simulink model "IEEE33BusTestSystem_DG_Control_IMC"  (R2019a)
settings: Solver=ode23t  StartTime=0.0  StopTime=20  FixedStep=5e-5  RelTol=1e-3
values from neighbouring files (symbols this model uses):
  du_n = 500    [IEEE33BusSystem_Control_Sim.m]    (also in IEEE33BusSystem_Control_Sim_nq3.m; IEEE33BusSystem_Control_Sim_nq5.m; IEEE33BusSystem_Ident.m; IEEE33BusSystem_Sim_compare.m)
  dy_n = 0.03    [IEEE33BusSystem_Control_Sim.m]    (also in IEEE33BusSystem_Control_Sim_nq3.m; IEEE33BusSystem_Control_Sim_nq5.m; IEEE33BusSystem_Ident.m; IEEE33BusSystem_Sim_compare.m)
  P_dg0 = 300*ones(1,6)    [IEEE33BusSystem_Control_Sim.m]    (also in IEEE33BusSystem_Control_Sim_nq3.m; IEEE33BusSystem_Control_Sim_nq5.m; IEEE33BusSystem_Ident.m; IEEE33BusSystem_op.m)
  P_dgf = 100*ones(1,6)    [IEEE33BusSystem_Control_Sim.m]    (also in IEEE33BusSystem_Control_Sim_nq3.m; IEEE33BusSystem_Control_Sim_nq5.m; IEEE33BusSystem_op.m = 300*ones(1,6); Kimc_d1_sce1-0.mat = [100 100 100 100 100 100])
  Q_dg0 = zeros(1,6)    [IEEE33BusSystem_Control_Sim.m]    (also in IEEE33BusSystem_Control_Sim_nq3.m; IEEE33BusSystem_Control_Sim_nq5.m; IEEE33BusSystem_Ident.m; IEEE33BusSystem_op.m)
  Tp = 500e-3    (= 0.5)    [IEEE33BusSystem.m]    (also in Kimc_d1_sce1-0.mat = 0.05; Kimc_d1_sce1-1.mat = 0.05; Kimc_d1_sce1-2.mat = 0.05; Kimc_d1_sce1-3.mat = 0.05)
  tPdg = 10*ones(1,6)    [IEEE33BusSystem_Control_Sim.m]    (also in IEEE33BusSystem_Control_Sim_nq3.m; IEEE33BusSystem_Control_Sim_nq5.m; IEEE33BusSystem_op.m = 0.5*ones(1,6); Kimc_d1_sce1-0.mat = [10 10 10 10 10 10])
  Tq = 50e-3    (= 0.05)    [IEEE33BusSystem.m]    (also in Kimc_d1_sce1-0.mat; Kimc_d1_sce1-1.mat; Kimc_d1_sce1-2.mat; Kimc_d1_sce1-3.mat)
  Ts = 0.005    [IEEE33BusSystem_Control_Sim.m]    (also in IEEE33BusSystem_Control_Sim_nq3.m; IEEE33BusSystem_Control_Sim_nq5.m; IEEE33BusSystem_Sim_compare.m = tout_d(2)-tout_d(1); IEEE33BusSystem_op.m)
  tsp = 3*ones(1,6)    [IEEE33BusSystem_Control_Sim.m]    (also in IEEE33BusSystem_Control_Sim_nq3.m; IEEE33BusSystem_Control_Sim_nq5.m; Kimc_d1_sce1-0.mat = [3 3 3 3 3 3]; Kimc_d1_sce1-1.mat = [3 3 3 3 3 3])
  v0 = ones(1,33)    [IEEE33BusSystem_Control_Sim.m]    (also in IEEE33BusSystem_Control_Sim_nq3.m; IEEE33BusSystem_Control_Sim_nq5.m; IEEE33BusSystem_Ident.m; IEEE33BusSystem_op.m)
  V_0 = v0_sim(CVs_sel)    [IEEE33BusSystem_Control_Sim.m]    (also in IEEE33BusSystem_Control_Sim_nq3.m = [v0_sim(14), v0_sim(18), v0_sim(21), v0_sim(25), v0_sim(30),; IEEE33BusSystem_Control_Sim_nq5.m = [v0_sim(14), v0_sim(18), v0_sim(21), v0_sim(25), v0_sim(30),; IEEE33BusSystem_Ident.m; IEEE33BusSystem_op.m = [v0(14), v0(18), v0(21), v0(25), v0(30), v0(33)])
  Vsp = V_0    [IEEE33BusSystem_Control_Sim.m]    (also in IEEE33BusSystem_Control_Sim_nq3.m; IEEE33BusSystem_Control_Sim_nq5.m; Kimc_d1_sce1-0.mat = [0.9549 0.956 0.9966 0.9787 0.9486 0.9462]; Kimc_d1_sce1-1.mat = [0.9549 0.956 0.9966 0.9787 0.9486 0.9462])
libraries: powerlib x160, powerlib_meascontrol x33, cstblocks x2
(part 2 of 4)

== system IEEE33BusTestSystem_DG_Control_IMC/ADN/Bus_13 ==
  Bus Load 13 : powerlib/Elements/Three-Phase Series RLC Load  LConnTagsString=A|B|C  Configuration=Y (grounded)  NominalVoltage=(12660)*v0(13)  Vabc=[1e3 1e3 1e3]  Vabcp=[1e3 1e3 1e3]  NominalFrequency=50  UnbalancedPower=off  ActivePower=60e3  InductivePower=35e3  CapacitivePower=0  Pabc=[10e3 9e3 11e3]  QLabc=[100 90 110]  QCabc=[100 90 110]  Pabcp=[10e3 9e3 11e3]  QLabcp=[100 90 110]  QCabcp=[100 90 110]  Measurements=None  LoadType=constant PQ
      settings: SourceProductName=Simscape Electrical
  Bus_13 : powerlib/Measurements/Three-Phase V-I Measurement  VoltageMeasurement=phase-to-phase  SetLabelV=on  LabelV=v13_pu  Vpu=off  VpuLL=on  CurrentMeasurement=yes  SetLabelI=on  LabelI=I1213_pu  Ipu=off  Pbase=100e6  Vbase=12660  OutputType=Complex  PhasorSimulation=on  PSBequivalent=0
      settings: SourceProductName=Simscape Electrical
  CB3-2 : powerlib/Elements/Three-Phase Breaker  InitialState=open  SwitchA=on  SwitchB=on  SwitchC=on  SwitchTimes="[1/60  5/60]"  External=on  BreakerResistance=0.01  SnubberResistance=1e6  SnubberCapacitance=inf  Measurements=None
      settings: SourceProductName=Simscape Electrical
  InPhaseA : PMIOPort  Side=Left
  InPhaseB : PMIOPort  Port=2  Side=Left
  InPhaseC : PMIOPort  Port=3  Side=Left
  OutPhaseA : PMIOPort  Port=4  Side=Right
  OutPhaseB : PMIOPort  Port=5  Side=Right
  OutPhaseC : PMIOPort  Port=6  Side=Right
  wires:
  [CB13to14] -> CB3-2/1
  connections:
  Bus Load 13/LConn1 -- CB3-2/LConn1 -- Bus_13/RConn1
  CB3-2/RConn3 -- OutPhaseC/RConn1
  Bus Load 13/LConn2 -- CB3-2/LConn2 -- Bus_13/RConn2
  Bus_13/RConn3 -- CB3-2/LConn3 -- Bus Load 13/LConn3
  CB3-2/RConn1 -- OutPhaseA/RConn1
  CB3-2/RConn2 -- OutPhaseB/RConn1
  InPhaseB/RConn1 -- Bus_13/LConn2
  Bus_13/LConn1 -- InPhaseA/RConn1
  InPhaseC/RConn1 -- Bus_13/LConn3

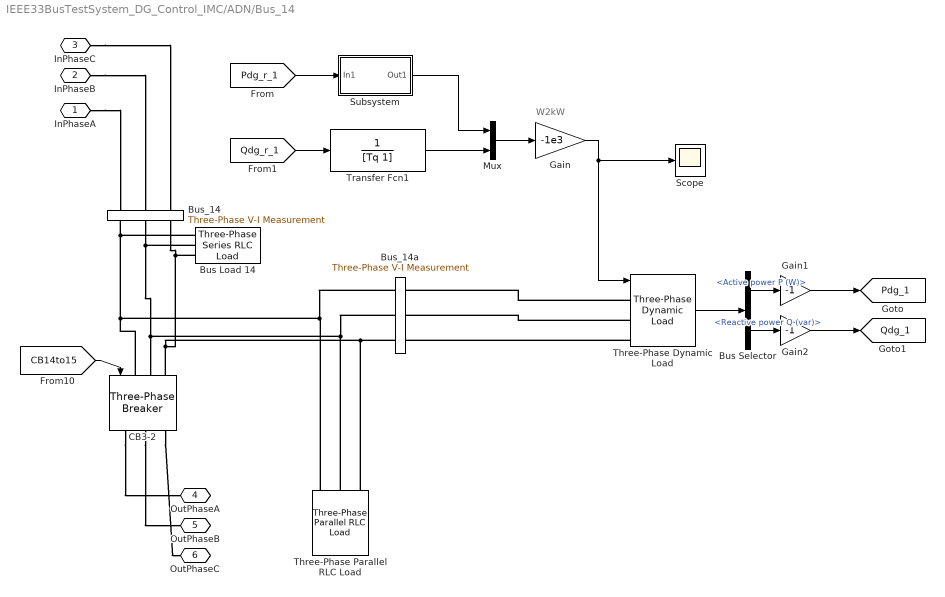
== system IEEE33BusTestSystem_DG_Control_IMC/ADN/Bus_14 ==
  note: W2kW
  Bus Load 14 : powerlib/Elements/Three-Phase Series RLC Load  LConnTagsString=A|B|C  Configuration=Y (grounded)  NominalVoltage=(12660)*v0(14)  Vabc=[1e3 1e3 1e3]  Vabcp=[1e3 1e3 1e3]  NominalFrequency=50  UnbalancedPower=off  ActivePower=120e3  InductivePower=80e3  CapacitivePower=0  Pabc=[10e3 9e3 11e3]  QLabc=[100 90 110]  QCabc=[100 90 110]  Pabcp=[10e3 9e3 11e3]  QLabcp=[100 90 110]  QCabcp=[100 90 110]  Measurements=None  LoadType=constant PQ
      settings: SourceProductName=Simscape Electrical
  Bus Selector : BusSelector  OutputSignals=Active power P (W),Reactive power Q (var)
  Bus_14 : powerlib/Measurements/Three-Phase V-I Measurement  VoltageMeasurement=phase-to-phase  SetLabelV=on  LabelV=v14_pu  Vpu=off  VpuLL=on  CurrentMeasurement=yes  SetLabelI=on  LabelI=I1314_pu  Ipu=off  Pbase=100e6  Vbase=12660  OutputType=Complex  PhasorSimulation=on  PSBequivalent=0
      settings: SourceProductName=Simscape Electrical
  Bus_14a : powerlib/Measurements/Three-Phase V-I Measurement  VoltageMeasurement=no  SetLabelV=off  LabelV=v14a_pu  Vpu=off  VpuLL=off  CurrentMeasurement=yes  SetLabelI=on  LabelI=I14a_pu  Ipu=off  Pbase=100e6  Vbase=500e3  OutputType=Complex  PhasorSimulation=on  PSBequivalent=0
      settings: SourceProductName=Simscape Electrical
  CB3-2 : powerlib/Elements/Three-Phase Breaker  InitialState=open  SwitchA=on  SwitchB=on  SwitchC=on  SwitchTimes="[1/60  5/60]"  External=on  BreakerResistance=0.01  SnubberResistance=1e6  SnubberCapacitance=inf  Measurements=None
      settings: SourceProductName=Simscape Electrical
  Gain : Gain  Gain=-1e3
  Gain1 : Gain  Gain=-1
  Gain2 : Gain  Gain=-1
  Mux : Mux  Inputs=2
  Scope : Scope
  Subsystem : Subsystem
  Three-Phase Dynamic Load : powerlib/Elements/Three-Phase Dynamic Load  NominalVoltage=[ 12660 50 ]  ActiveReactivePowers=[-P_dg0(1) Q_dg0(1)]*1e3  PositiveSequence=[V_0(1) 0]  ExternalControl=on  NpNq=[1.3 2]  TimeConstants="[0  0  0  0]"  MinimumVoltage=0.7  Tfilter=1e-4  LoadFlowParameters=[4,0,0,0,0]
      settings: SourceProductName=Simscape Electrical  SourceProductBaseCode=PS
  Three-Phase Parallel RLC Load : powerlib/Elements/Three-Phase Parallel RLC Load  LConnTagsString=A|B|C  Configuration=Y (grounded)  NominalVoltage=12660  Vabc=[1e3 1e3 1e3]  Vabcp=[1e3 1e3 1e3]  NominalFrequency=50  UnbalancedPower=off  ActivePower=0.01  InductivePower=0  CapacitivePower=0  Pabc=[10e3 9e3 11e3]  QLabc=[100 90 110]  QCabc=[100 90 110]  Pabcp=[10e3 9e3 11e3]  QLabcp=[100 90 110]  QCabcp=[100 90 110]  Measurements=None  LoadType=constant Z
      settings: SourceProductName=Simscape Electrical
  Transfer Fcn1 : TransferFcn  Denominator=[Tq 1]
  InPhaseA : PMIOPort  Side=Left
  InPhaseB : PMIOPort  Port=2  Side=Left
  InPhaseC : PMIOPort  Port=3  Side=Left
  OutPhaseA : PMIOPort  Port=4  Side=Right
  OutPhaseB : PMIOPort  Port=5  Side=Right
  OutPhaseC : PMIOPort  Port=6  Side=Right
  tag scope: Pdg_1=global, Qdg_1=global
  wires:
  [CB14to15] -> CB3-2/1
  Mux/1 -> Gain/1
  Gain/1 -> Three-Phase Dynamic Load/1, Scope/1
  Three-Phase Dynamic Load/1 -> Bus Selector/1
  Subsystem/1(Out1) -> Mux/1
  Bus Selector/1 -> Gain1/1  "<Active power P (W)>"
  Bus Selector/2 -> Gain2/1  "<Reactive power Q (var)>"
  Gain1/1 -> [Pdg_1]
  Gain2/1 -> [Qdg_1]
  [Pdg_r_1] -> Subsystem/1(In1)
  [Qdg_r_1] -> Transfer Fcn1/1
  Transfer Fcn1/1 -> Mux/2
  connections:
  CB3-2/LConn1 -- Three-Phase Parallel RLC Load/LConn1 -- Bus_14a/RConn1 -- Bus Load 14/LConn1 -- Bus_14/RConn1
  CB3-2/RConn3 -- OutPhaseC/RConn1
  Bus_14/RConn3 -- Bus_14a/RConn3 -- Three-Phase Parallel RLC Load/LConn3 -- CB3-2/LConn3 -- Bus Load 14/LConn3
  CB3-2/RConn1 -- OutPhaseA/RConn1
  CB3-2/RConn2 -- OutPhaseB/RConn1
  InPhaseB/RConn1 -- Bus_14/LConn2
  InPhaseA/RConn1 -- Bus_14/LConn1
  InPhaseC/RConn1 -- Bus_14/LConn3
  Bus_14/RConn2 -- Bus Load 14/LConn2 -- Three-Phase Parallel RLC Load/LConn2 -- Bus_14a/RConn2 -- CB3-2/LConn2
  Three-Phase Dynamic Load/LConn1 -- Bus_14a/LConn1
  Three-Phase Dynamic Load/LConn2 -- Bus_14a/LConn2
  Three-Phase Dynamic Load/LConn3 -- Bus_14a/LConn3

== system IEEE33BusTestSystem_DG_Control_IMC/ADN/Bus_15 ==
  Bus Load 15 : powerlib/Elements/Three-Phase Series RLC Load  LConnTagsString=A|B|C  Configuration=Y (grounded)  NominalVoltage=(12660)*v0(15)  Vabc=[1e3 1e3 1e3]  Vabcp=[1e3 1e3 1e3]  NominalFrequency=50  UnbalancedPower=off  ActivePower=60e3  InductivePower=10e3  CapacitivePower=0  Pabc=[10e3 9e3 11e3]  QLabc=[100 90 110]  QCabc=[100 90 110]  Pabcp=[10e3 9e3 11e3]  QLabcp=[100 90 110]  QCabcp=[100 90 110]  Measurements=None  LoadType=constant PQ
      settings: SourceProductName=Simscape Electrical
  Bus_15 : powerlib/Measurements/Three-Phase V-I Measurement  VoltageMeasurement=phase-to-phase  SetLabelV=on  LabelV=v15_pu  Vpu=off  VpuLL=on  CurrentMeasurement=yes  SetLabelI=on  LabelI=I1415_pu  Ipu=off  Pbase=100e6  Vbase=12660  OutputType=Complex  PhasorSimulation=on  PSBequivalent=0
      settings: SourceProductName=Simscape Electrical
  CB3-2 : powerlib/Elements/Three-Phase Breaker  InitialState=open  SwitchA=on  SwitchB=on  SwitchC=on  SwitchTimes="[1/60  5/60]"  External=on  BreakerResistance=0.01  SnubberResistance=1e6  SnubberCapacitance=inf  Measurements=None
      settings: SourceProductName=Simscape Electrical
  InPhaseA : PMIOPort  Side=Left
  InPhaseB : PMIOPort  Port=2  Side=Left
  InPhaseC : PMIOPort  Port=3  Side=Left
  OutPhaseA : PMIOPort  Port=4  Side=Right
  OutPhaseB : PMIOPort  Port=5  Side=Right
  OutPhaseC : PMIOPort  Port=6  Side=Right
  InPhaseA1 : PMIOPort  Port=7  Side=Left
  InPhaseB1 : PMIOPort  Port=8  Side=Left
  InPhaseC1 : PMIOPort  Port=9  Side=Left
  wires:
  [CB15to16] -> CB3-2/1
  connections:
  Bus Load 15/LConn1 -- CB3-2/LConn1 -- Bus_15/RConn1
  CB3-2/RConn3 -- OutPhaseC/RConn1
  Bus Load 15/LConn2 -- CB3-2/LConn2 -- Bus_15/RConn2
  Bus Load 15/LConn3 -- CB3-2/LConn3 -- Bus_15/RConn3
  CB3-2/RConn1 -- OutPhaseA/RConn1
  CB3-2/RConn2 -- OutPhaseB/RConn1
  InPhaseA1/RConn1 -- InPhaseA/RConn1 -- Bus_15/LConn1
  InPhaseB1/RConn1 -- InPhaseB/RConn1 -- Bus_15/LConn2
  InPhaseC1/RConn1 -- InPhaseC/RConn1 -- Bus_15/LConn3

== system IEEE33BusTestSystem_DG_Control_IMC/ADN/Bus_16 ==
  Bus Load 16 : powerlib/Elements/Three-Phase Series RLC Load  LConnTagsString=A|B|C  Configuration=Y (grounded)  NominalVoltage=(12660)*v0(16)  Vabc=[1e3 1e3 1e3]  Vabcp=[1e3 1e3 1e3]  NominalFrequency=50  UnbalancedPower=off  ActivePower=60e3  InductivePower=20e3  CapacitivePower=0  Pabc=[10e3 9e3 11e3]  QLabc=[100 90 110]  QCabc=[100 90 110]  Pabcp=[10e3 9e3 11e3]  QLabcp=[100 90 110]  QCabcp=[100 90 110]  Measurements=None  LoadType=constant PQ
      settings: SourceProductName=Simscape Electrical
  Bus_16 : powerlib/Measurements/Three-Phase V-I Measurement  VoltageMeasurement=phase-to-phase  SetLabelV=on  LabelV=v16_pu  Vpu=off  VpuLL=on  CurrentMeasurement=yes  SetLabelI=on  LabelI=I1516_pu  Ipu=off  Pbase=100e6  Vbase=12660  OutputType=Complex  PhasorSimulation=on  PSBequivalent=0
      settings: SourceProductName=Simscape Electrical
  CB3-2 : powerlib/Elements/Three-Phase Breaker  InitialState=open  SwitchA=on  SwitchB=on  SwitchC=on  SwitchTimes="[1/60  5/60]"  External=on  BreakerResistance=0.01  SnubberResistance=1e6  SnubberCapacitance=inf  Measurements=None
      settings: SourceProductName=Simscape Electrical
  InPhaseA : PMIOPort  Side=Left
  InPhaseB : PMIOPort  Port=2  Side=Left
  InPhaseC : PMIOPort  Port=3  Side=Left
  OutPhaseA : PMIOPort  Port=4  Side=Right
  OutPhaseB : PMIOPort  Port=5  Side=Right
  OutPhaseC : PMIOPort  Port=6  Side=Right
  wires:
  [CB16to17] -> CB3-2/1
  connections:
  Bus_16/RConn1 -- CB3-2/LConn1 -- Bus Load 16/LConn1
  CB3-2/RConn3 -- OutPhaseC/RConn1
  Bus Load 16/LConn2 -- CB3-2/LConn2 -- Bus_16/RConn2
  Bus Load 16/LConn3 -- CB3-2/LConn3 -- Bus_16/RConn3
  CB3-2/RConn1 -- OutPhaseA/RConn1
  CB3-2/RConn2 -- OutPhaseB/RConn1
  InPhaseC/RConn1 -- Bus_16/LConn3
  InPhaseB/RConn1 -- Bus_16/LConn2
  InPhaseA/RConn1 -- Bus_16/LConn1

== system IEEE33BusTestSystem_DG_Control_IMC/ADN/Bus_17 ==
  Bus Load 17 : powerlib/Elements/Three-Phase Series RLC Load  LConnTagsString=A|B|C  Configuration=Y (grounded)  NominalVoltage=(12660)*v0(17)  Vabc=[1e3 1e3 1e3]  Vabcp=[1e3 1e3 1e3]  NominalFrequency=50  UnbalancedPower=off  ActivePower=60e3  InductivePower=20e3  CapacitivePower=0  Pabc=[10e3 9e3 11e3]  QLabc=[100 90 110]  QCabc=[100 90 110]  Pabcp=[10e3 9e3 11e3]  QLabcp=[100 90 110]  QCabcp=[100 90 110]  Measurements=None  LoadType=constant PQ
      settings: SourceProductName=Simscape Electrical
  Bus_17 : powerlib/Measurements/Three-Phase V-I Measurement  VoltageMeasurement=phase-to-phase  SetLabelV=on  LabelV=v17_pu  Vpu=off  VpuLL=on  CurrentMeasurement=yes  SetLabelI=on  LabelI=I1617_pu  Ipu=off  Pbase=100e6  Vbase=12660  OutputType=Complex  PhasorSimulation=on  PSBequivalent=0
      settings: SourceProductName=Simscape Electrical
  CB3-1 : powerlib/Elements/Three-Phase Breaker  InitialState=open  SwitchA=on  SwitchB=on  SwitchC=on  SwitchTimes="[1/60  5/60]"  External=on  BreakerResistance=0.01  SnubberResistance=1e6  SnubberCapacitance=inf  Measurements=None
      settings: SourceProductName=Simscape Electrical
  CB3-2 : powerlib/Elements/Three-Phase Breaker  InitialState=open  SwitchA=on  SwitchB=on  SwitchC=on  SwitchTimes="[1/60  5/60]"  External=on  BreakerResistance=0.01  SnubberResistance=1e6  SnubberCapacitance=inf  Measurements=None
      settings: SourceProductName=Simscape Electrical
  Step : Step  Time=2  Before=1  SampleTime=0
  InPhaseA : PMIOPort  Side=Left
  InPhaseB : PMIOPort  Port=2  Side=Left
  InPhaseC : PMIOPort  Port=3  Side=Left
  OutPhaseA : PMIOPort  Port=4  Side=Right
  OutPhaseB : PMIOPort  Port=5  Side=Right
  OutPhaseC : PMIOPort  Port=6  Side=Right
  wires:
  [CB17to18] -> CB3-2/1
  Step/1 -> CB3-1/1
  connections:
  CB3-2/LConn1 -- Bus_17/RConn1 -- CB3-1/RConn1
  CB3-2/RConn3 -- OutPhaseC/RConn1
  Bus_17/RConn2 -- CB3-1/RConn2 -- CB3-2/LConn2
  Bus_17/RConn3 -- CB3-1/RConn3 -- CB3-2/LConn3
  CB3-2/RConn1 -- OutPhaseA/RConn1
  CB3-2/RConn2 -- OutPhaseB/RConn1
  InPhaseA/RConn1 -- Bus_17/LConn1
  InPhaseB/RConn1 -- Bus_17/LConn2
  InPhaseC/RConn1 -- Bus_17/LConn3
  CB3-1/LConn1 -- Bus Load 17/LConn1
  CB3-1/LConn2 -- Bus Load 17/LConn2
  CB3-1/LConn3 -- Bus Load 17/LConn3

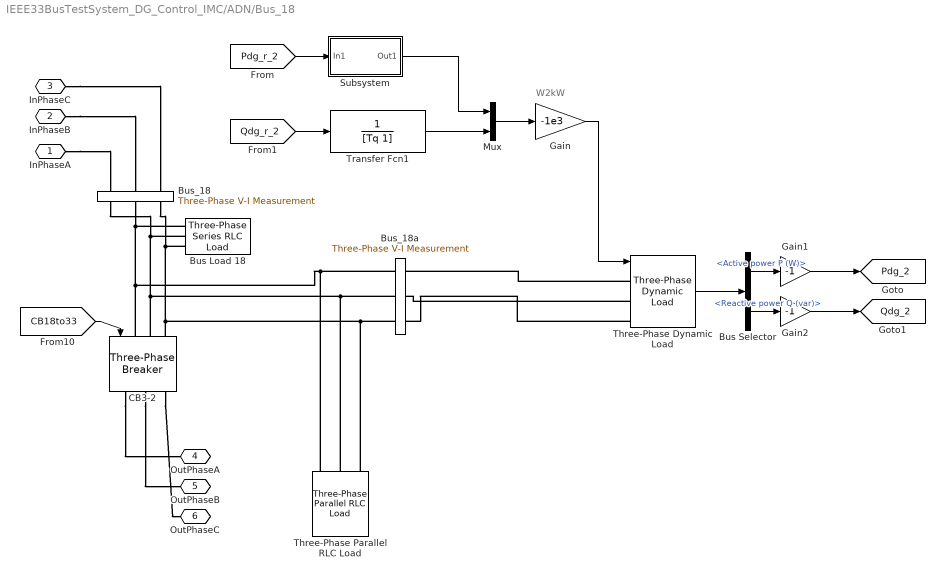
== system IEEE33BusTestSystem_DG_Control_IMC/ADN/Bus_18 ==
  note: W2kW
  Bus Load 18 : powerlib/Elements/Three-Phase Series RLC Load  LConnTagsString=A|B|C  Configuration=Y (grounded)  NominalVoltage=(12660)*v0(18)  Vabc=[1e3 1e3 1e3]  Vabcp=[1e3 1e3 1e3]  NominalFrequency=50  UnbalancedPower=off  ActivePower=90e3  InductivePower=40e3  CapacitivePower=0  Pabc=[10e3 9e3 11e3]  QLabc=[100 90 110]  QCabc=[100 90 110]  Pabcp=[10e3 9e3 11e3]  QLabcp=[100 90 110]  QCabcp=[100 90 110]  Measurements=None  LoadType=constant PQ
      settings: SourceProductName=Simscape Electrical
  Bus Selector : BusSelector  OutputSignals=Active power P (W),Reactive power Q (var)
  Bus_18 : powerlib/Measurements/Three-Phase V-I Measurement  VoltageMeasurement=phase-to-phase  SetLabelV=on  LabelV=v18_pu  Vpu=off  VpuLL=on  CurrentMeasurement=yes  SetLabelI=on  LabelI=I1718_pu  Ipu=off  Pbase=100e6  Vbase=12660  OutputType=Complex  PhasorSimulation=on  PSBequivalent=0
      settings: SourceProductName=Simscape Electrical
  Bus_18a : powerlib/Measurements/Three-Phase V-I Measurement  VoltageMeasurement=no  SetLabelV=off  LabelV=v14a_pu  Vpu=off  VpuLL=off  CurrentMeasurement=yes  SetLabelI=on  LabelI=I18a_pu  Ipu=off  Pbase=100e6  Vbase=500e3  OutputType=Complex  PhasorSimulation=on  PSBequivalent=0
      settings: SourceProductName=Simscape Electrical
  CB3-2 : powerlib/Elements/Three-Phase Breaker  InitialState=open  SwitchA=on  SwitchB=on  SwitchC=on  SwitchTimes="[1/60  5/60]"  External=on  BreakerResistance=0.01  SnubberResistance=1e6  SnubberCapacitance=inf  Measurements=None
      settings: SourceProductName=Simscape Electrical
  Gain : Gain  Gain=-1e3
  Gain1 : Gain  Gain=-1
  Gain2 : Gain  Gain=-1
  Mux : Mux  Inputs=2
  Subsystem : Subsystem
  Three-Phase Dynamic Load : powerlib/Elements/Three-Phase Dynamic Load  NominalVoltage=[ 12660 50 ]  ActiveReactivePowers=[-P_dg0(2) Q_dg0(2)]*1e3  PositiveSequence=[V_0(2) 0]  ExternalControl=on  NpNq=[1.3 2]  TimeConstants="[0  0  0  0]"  MinimumVoltage=0.7  Tfilter=1e-4  LoadFlowParameters=[4,0,0,0,0]
      settings: SourceProductName=Simscape Electrical  SourceProductBaseCode=PS
  Three-Phase Parallel RLC Load : powerlib/Elements/Three-Phase Parallel RLC Load  LConnTagsString=A|B|C  Configuration=Y (grounded)  NominalVoltage=12660  Vabc=[1e3 1e3 1e3]  Vabcp=[1e3 1e3 1e3]  NominalFrequency=50  UnbalancedPower=off  ActivePower=0.01  InductivePower=0  CapacitivePower=0  Pabc=[10e3 9e3 11e3]  QLabc=[100 90 110]  QCabc=[100 90 110]  Pabcp=[10e3 9e3 11e3]  QLabcp=[100 90 110]  QCabcp=[100 90 110]  Measurements=None  LoadType=constant Z
      settings: SourceProductName=Simscape Electrical
  Transfer Fcn1 : TransferFcn  Denominator=[Tq 1]
  InPhaseA : PMIOPort  Side=Left
  InPhaseB : PMIOPort  Port=2  Side=Left
  InPhaseC : PMIOPort  Port=3  Side=Left
  OutPhaseA : PMIOPort  Port=4  Side=Right
  OutPhaseB : PMIOPort  Port=5  Side=Right
  OutPhaseC : PMIOPort  Port=6  Side=Right
  tag scope: Pdg_2=global, Qdg_2=global
  wires:
  [CB18to33] -> CB3-2/1
  Subsystem/1(Out1) -> Mux/1
  Bus Selector/1 -> Gain1/1  "<Active power P (W)>"
  [Pdg_r_2] -> Subsystem/1(In1)
  Gain2/1 -> [Qdg_2]
  Bus Selector/2 -> Gain2/1  "<Reactive power Q (var)>"
  Mux/1 -> Gain/1
  Three-Phase Dynamic Load/1 -> Bus Selector/1
  Gain/1 -> Three-Phase Dynamic Load/1
  Gain1/1 -> [Pdg_2]
  [Qdg_r_2] -> Transfer Fcn1/1
  Transfer Fcn1/1 -> Mux/2
  connections:
  Bus_18/RConn1 -- Three-Phase Parallel RLC Load/LConn1 -- Bus_18a/RConn1 -- CB3-2/LConn1 -- Bus Load 18/LConn1
  CB3-2/RConn3 -- OutPhaseC/RConn1
  Bus Load 18/LConn2 -- Three-Phase Parallel RLC Load/LConn2 -- Bus_18a/RConn2 -- CB3-2/LConn2 -- Bus_18/RConn2
  Bus Load 18/LConn3 -- Three-Phase Parallel RLC Load/LConn3 -- Bus_18a/RConn3 -- CB3-2/LConn3 -- Bus_18/RConn3
  CB3-2/RConn1 -- OutPhaseA/RConn1
  CB3-2/RConn2 -- OutPhaseB/RConn1
  InPhaseA/RConn1 -- Bus_18/LConn1
  InPhaseB/RConn1 -- Bus_18/LConn2
  InPhaseC/RConn1 -- Bus_18/LConn3
  Three-Phase Dynamic Load/LConn1 -- Bus_18a/LConn1
  Three-Phase Dynamic Load/LConn3 -- Bus_18a/LConn3
  Three-Phase Dynamic Load/LConn2 -- Bus_18a/LConn2

== system IEEE33BusTestSystem_DG_Control_IMC/ADN/Bus_19 ==
  Bus Load 19 : powerlib/Elements/Three-Phase Series RLC Load  LConnTagsString=A|B|C  Configuration=Y (grounded)  NominalVoltage=(12660)*v0(19)  Vabc=[1e3 1e3 1e3]  Vabcp=[1e3 1e3 1e3]  NominalFrequency=50  UnbalancedPower=off  ActivePower=90e3  InductivePower=40e3  CapacitivePower=0  Pabc=[10e3 9e3 11e3]  QLabc=[100 90 110]  QCabc=[100 90 110]  Pabcp=[10e3 9e3 11e3]  QLabcp=[100 90 110]  QCabcp=[100 90 110]  Measurements=None  LoadType=constant PQ
      settings: SourceProductName=Simscape Electrical
  Bus_19 : powerlib/Measurements/Three-Phase V-I Measurement  VoltageMeasurement=phase-to-phase  SetLabelV=on  LabelV=v19_pu  Vpu=off  VpuLL=on  CurrentMeasurement=yes  SetLabelI=on  LabelI=I219_pu  Ipu=off  Pbase=100e6  Vbase=12660  OutputType=Complex  PhasorSimulation=on  PSBequivalent=0
      settings: SourceProductName=Simscape Electrical
  CB3-2 : powerlib/Elements/Three-Phase Breaker  InitialState=open  SwitchA=on  SwitchB=on  SwitchC=on  SwitchTimes="[1/60  5/60]"  External=on  BreakerResistance=0.01  SnubberResistance=1e6  SnubberCapacitance=inf  Measurements=None
      settings: SourceProductName=Simscape Electrical
  InPhaseA : PMIOPort  Side=Left
  InPhaseB : PMIOPort  Port=2  Side=Left
  InPhaseC : PMIOPort  Port=3  Side=Left
  OutPhaseA : PMIOPort  Port=4  Side=Right
  OutPhaseB : PMIOPort  Port=5  Side=Right
  OutPhaseC : PMIOPort  Port=6  Side=Right
  wires:
  [CB19to20] -> CB3-2/1
  connections:
  Bus_19/RConn1 -- CB3-2/LConn1 -- Bus Load 19/LConn1
  CB3-2/RConn3 -- OutPhaseC/RConn1
  Bus Load 19/LConn2 -- CB3-2/LConn2 -- Bus_19/RConn2
  Bus_19/RConn3 -- CB3-2/LConn3 -- Bus Load 19/LConn3
  CB3-2/RConn1 -- OutPhaseA/RConn1
  CB3-2/RConn2 -- OutPhaseB/RConn1
  Bus_19/LConn1 -- InPhaseA/RConn1
  InPhaseB/RConn1 -- Bus_19/LConn2
  InPhaseC/RConn1 -- Bus_19/LConn3

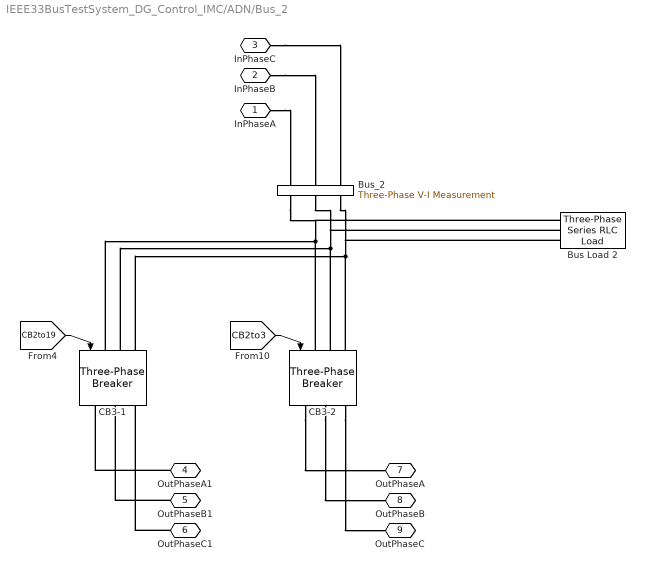
== system IEEE33BusTestSystem_DG_Control_IMC/ADN/Bus_2 ==
  Bus Load 2 : powerlib/Elements/Three-Phase Series RLC Load  LConnTagsString=A|B|C  Configuration=Y (grounded)  NominalVoltage=(12660)*v0(2)  Vabc=[1e3 1e3 1e3]  Vabcp=[1e3 1e3 1e3]  NominalFrequency=50  UnbalancedPower=off  ActivePower=100e3  InductivePower=60e3  CapacitivePower=0  Pabc=[10e3 9e3 11e3]  QLabc=[100 90 110]  QCabc=[100 90 110]  Pabcp=[10e3 9e3 11e3]  QLabcp=[100 90 110]  QCabcp=[100 90 110]  Measurements=None  LoadType=constant PQ
      settings: SourceProductName=Simscape Electrical
  Bus_2 : powerlib/Measurements/Three-Phase V-I Measurement  VoltageMeasurement=phase-to-phase  SetLabelV=on  LabelV=v2_pu  Vpu=off  VpuLL=on  CurrentMeasurement=yes  SetLabelI=on  LabelI=I12_pu  Ipu=off  Pbase=10e6  Vbase=12660  OutputType=Complex  PhasorSimulation=on  PSBequivalent=0
      settings: SourceProductName=Simscape Electrical
  CB3-1 : powerlib/Elements/Three-Phase Breaker  InitialState=open  SwitchA=on  SwitchB=on  SwitchC=on  SwitchTimes="[1/60  5/60]"  External=on  BreakerResistance=0.01  SnubberResistance=1e6  SnubberCapacitance=inf  Measurements=None
      settings: SourceProductName=Simscape Electrical
  CB3-2 : powerlib/Elements/Three-Phase Breaker  InitialState=open  SwitchA=on  SwitchB=on  SwitchC=on  SwitchTimes="[1/60  5/60]"  External=on  BreakerResistance=0.01  SnubberResistance=1e6  SnubberCapacitance=inf  Measurements=None
      settings: SourceProductName=Simscape Electrical
  InPhaseA : PMIOPort  Side=Left
  InPhaseB : PMIOPort  Port=2  Side=Left
  InPhaseC : PMIOPort  Port=3  Side=Left
  OutPhaseA1 : PMIOPort  Port=4  Side=Right
  OutPhaseB1 : PMIOPort  Port=5  Side=Right
  OutPhaseC1 : PMIOPort  Port=6  Side=Right
  OutPhaseA : PMIOPort  Port=7  Side=Right
  OutPhaseB : PMIOPort  Port=8  Side=Right
  OutPhaseC : PMIOPort  Port=9  Side=Right
  wires:
  [CB2to3] -> CB3-2/1
  [CB2to19] -> CB3-1/1
  connections:
  CB3-1/LConn1 -- CB3-2/LConn1 -- Bus Load 2/LConn1 -- Bus_2/RConn1
  CB3-1/LConn2 -- Bus_2/RConn2 -- Bus Load 2/LConn2 -- CB3-2/LConn2
  CB3-1/LConn3 -- Bus_2/RConn3 -- Bus Load 2/LConn3 -- CB3-2/LConn3
  InPhaseC/RConn1 -- Bus_2/LConn3
  InPhaseB/RConn1 -- Bus_2/LConn2
  InPhaseA/RConn1 -- Bus_2/LConn1
  OutPhaseA1/RConn1 -- CB3-1/RConn1
  OutPhaseC1/RConn1 -- CB3-1/RConn3
  OutPhaseB1/RConn1 -- CB3-1/RConn2
  CB3-2/RConn1 -- OutPhaseA/RConn1
  CB3-2/RConn2 -- OutPhaseB/RConn1
  CB3-2/RConn3 -- OutPhaseC/RConn1

== system IEEE33BusTestSystem_DG_Control_IMC/ADN/Bus_20 ==
  Bus Load 20 : powerlib/Elements/Three-Phase Series RLC Load  LConnTagsString=A|B|C  Configuration=Y (grounded)  NominalVoltage=(12660)*v0(20)  Vabc=[1e3 1e3 1e3]  Vabcp=[1e3 1e3 1e3]  NominalFrequency=50  UnbalancedPower=off  ActivePower=90e3  InductivePower=40e3  CapacitivePower=0  Pabc=[10e3 9e3 11e3]  QLabc=[100 90 110]  QCabc=[100 90 110]  Pabcp=[10e3 9e3 11e3]  QLabcp=[100 90 110]  QCabcp=[100 90 110]  Measurements=None  LoadType=constant PQ
      settings: SourceProductName=Simscape Electrical
  Bus_20 : powerlib/Measurements/Three-Phase V-I Measurement  VoltageMeasurement=phase-to-phase  SetLabelV=on  LabelV=v20_pu  Vpu=off  VpuLL=on  CurrentMeasurement=yes  SetLabelI=on  LabelI=I1920_pu  Ipu=off  Pbase=100e6  Vbase=12660  OutputType=Complex  PhasorSimulation=on  PSBequivalent=0
      settings: SourceProductName=Simscape Electrical
  CB3-2 : powerlib/Elements/Three-Phase Breaker  InitialState=open  SwitchA=on  SwitchB=on  SwitchC=on  SwitchTimes="[1/60  5/60]"  External=on  BreakerResistance=0.01  SnubberResistance=1e6  SnubberCapacitance=inf  Measurements=None
      settings: SourceProductName=Simscape Electrical
  InPhaseA : PMIOPort  Side=Left
  InPhaseB : PMIOPort  Port=2  Side=Left
  InPhaseC : PMIOPort  Port=3  Side=Left
  OutPhaseA : PMIOPort  Port=4  Side=Right
  OutPhaseB : PMIOPort  Port=5  Side=Right
  OutPhaseC : PMIOPort  Port=6  Side=Right
  wires:
  [CB20to21] -> CB3-2/1
  connections:
  Bus_20/RConn1 -- CB3-2/LConn1 -- Bus Load 20/LConn1
  CB3-2/RConn3 -- OutPhaseC/RConn1
  Bus Load 20/LConn2 -- CB3-2/LConn2 -- Bus_20/RConn2
  Bus_20/RConn3 -- CB3-2/LConn3 -- Bus Load 20/LConn3
  CB3-2/RConn1 -- OutPhaseA/RConn1
  CB3-2/RConn2 -- OutPhaseB/RConn1
  InPhaseA/RConn1 -- Bus_20/LConn1
  InPhaseB/RConn1 -- Bus_20/LConn2
  InPhaseC/RConn1 -- Bus_20/LConn3

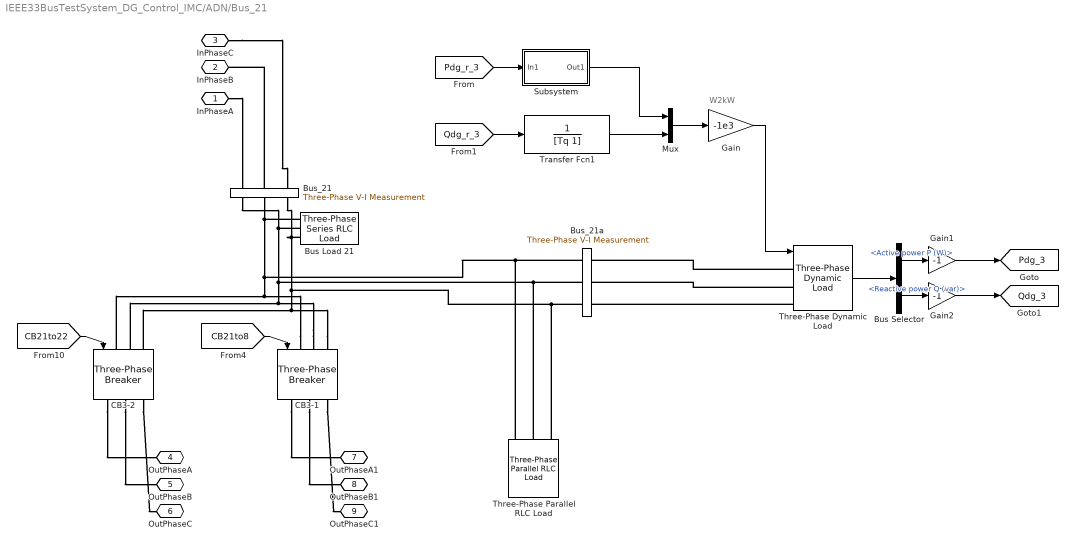
== system IEEE33BusTestSystem_DG_Control_IMC/ADN/Bus_21 ==
  note: W2kW
  Bus Load 21 : powerlib/Elements/Three-Phase Series RLC Load  LConnTagsString=A|B|C  Configuration=Y (grounded)  NominalVoltage=(12660)*v0(21)  Vabc=[1e3 1e3 1e3]  Vabcp=[1e3 1e3 1e3]  NominalFrequency=50  UnbalancedPower=off  ActivePower=90e3  InductivePower=40e3  CapacitivePower=0  Pabc=[10e3 9e3 11e3]  QLabc=[100 90 110]  QCabc=[100 90 110]  Pabcp=[10e3 9e3 11e3]  QLabcp=[100 90 110]  QCabcp=[100 90 110]  Measurements=None  LoadType=constant PQ
      settings: SourceProductName=Simscape Electrical
  Bus Selector : BusSelector  OutputSignals=Active power P (W),Reactive power Q (var)
  Bus_21 : powerlib/Measurements/Three-Phase V-I Measurement  VoltageMeasurement=phase-to-phase  SetLabelV=on  LabelV=v21_pu  Vpu=off  VpuLL=on  CurrentMeasurement=yes  SetLabelI=on  LabelI=I2021_pu  Ipu=off  Pbase=100e6  Vbase=12660  OutputType=Complex  PhasorSimulation=on  PSBequivalent=0
      settings: SourceProductName=Simscape Electrical
  Bus_21a : powerlib/Measurements/Three-Phase V-I Measurement  VoltageMeasurement=no  SetLabelV=off  LabelV=v14a_pu  Vpu=off  VpuLL=off  CurrentMeasurement=yes  SetLabelI=on  LabelI=I21a_pu  Ipu=off  Pbase=100e6  Vbase=500e3  OutputType=Complex  PhasorSimulation=on  PSBequivalent=0
      settings: SourceProductName=Simscape Electrical
  CB3-1 : powerlib/Elements/Three-Phase Breaker  InitialState=open  SwitchA=on  SwitchB=on  SwitchC=on  SwitchTimes="[1/60  5/60]"  External=on  BreakerResistance=0.01  SnubberResistance=1e6  SnubberCapacitance=inf  Measurements=None
      settings: SourceProductName=Simscape Electrical
  CB3-2 : powerlib/Elements/Three-Phase Breaker  InitialState=open  SwitchA=on  SwitchB=on  SwitchC=on  SwitchTimes="[1/60  5/60]"  External=on  BreakerResistance=0.01  SnubberResistance=1e6  SnubberCapacitance=inf  Measurements=None
      settings: SourceProductName=Simscape Electrical
  Gain : Gain  Gain=-1e3
  Gain1 : Gain  Gain=-1
  Gain2 : Gain  Gain=-1
  Mux : Mux  Inputs=2
  Subsystem : Subsystem
  Three-Phase Dynamic Load : powerlib/Elements/Three-Phase Dynamic Load  NominalVoltage=[ 12660 50 ]  ActiveReactivePowers=[-P_dg0(3) Q_dg0(3)]*1e3  PositiveSequence=[V_0(3) 0]  ExternalControl=on  NpNq=[1.3 2]  TimeConstants="[0  0  0  0]"  MinimumVoltage=0.7  Tfilter=1e-4  LoadFlowParameters=[4,0,0,0,0]
      settings: SourceProductName=Simscape Electrical  SourceProductBaseCode=PS
  Three-Phase Parallel RLC Load : powerlib/Elements/Three-Phase Parallel RLC Load  LConnTagsString=A|B|C  Configuration=Y (grounded)  NominalVoltage=12660  Vabc=[1e3 1e3 1e3]  Vabcp=[1e3 1e3 1e3]  NominalFrequency=50  UnbalancedPower=off  ActivePower=0.01  InductivePower=0  CapacitivePower=0  Pabc=[10e3 9e3 11e3]  QLabc=[100 90 110]  QCabc=[100 90 110]  Pabcp=[10e3 9e3 11e3]  QLabcp=[100 90 110]  QCabcp=[100 90 110]  Measurements=None  LoadType=constant Z
      settings: SourceProductName=Simscape Electrical
  Transfer Fcn1 : TransferFcn  Denominator=[Tq 1]
  InPhaseA : PMIOPort  Side=Left
  InPhaseB : PMIOPort  Port=2  Side=Left
  InPhaseC : PMIOPort  Port=3  Side=Left
  OutPhaseA : PMIOPort  Port=4  Side=Right
  OutPhaseB : PMIOPort  Port=5  Side=Right
  OutPhaseC : PMIOPort  Port=6  Side=Right
  OutPhaseA1 : PMIOPort  Port=7  Side=Right
  OutPhaseB1 : PMIOPort  Port=8  Side=Right
  OutPhaseC1 : PMIOPort  Port=9  Side=Right
  tag scope: Pdg_3=global, Qdg_3=global
  wires:
  [CB21to22] -> CB3-2/1
  [CB21to8] -> CB3-1/1
  Subsystem/1(Out1) -> Mux/1
  Transfer Fcn1/1 -> Mux/2
  Bus Selector/1 -> Gain1/1  "<Active power P (W)>"
  [Pdg_r_3] -> Subsystem/1(In1)
  Gain2/1 -> [Qdg_3]
  Bus Selector/2 -> Gain2/1  "<Reactive power Q (var)>"
  Mux/1 -> Gain/1
  Three-Phase Dynamic Load/1 -> Bus Selector/1
  Gain/1 -> Three-Phase Dynamic Load/1
  Gain1/1 -> [Pdg_3]
  [Qdg_r_3] -> Transfer Fcn1/1
  connections:
  CB3-1/LConn1 -- Three-Phase Parallel RLC Load/LConn1 -- Bus_21a/RConn1 -- Bus Load 21/LConn1 -- Bus_21/RConn1 -- CB3-2/LConn1
  CB3-2/RConn3 -- OutPhaseC/RConn1
  CB3-1/LConn2 -- Three-Phase Parallel RLC Load/LConn2 -- Bus_21a/RConn2 -- Bus Load 21/LConn2 -- Bus_21/RConn2 -- CB3-2/LConn2
  CB3-1/LConn3 -- Three-Phase Parallel RLC Load/LConn3 -- Bus_21a/RConn3 -- Bus_21/RConn3 -- Bus Load 21/LConn3 -- CB3-2/LConn3
  CB3-2/RConn1 -- OutPhaseA/RConn1
  CB3-2/RConn2 -- OutPhaseB/RConn1
  InPhaseA/RConn1 -- Bus_21/LConn1
  Bus_21/LConn2 -- InPhaseB/RConn1
  InPhaseC/RConn1 -- Bus_21/LConn3
  CB3-1/RConn3 -- OutPhaseC1/RConn1
  CB3-1/RConn1 -- OutPhaseA1/RConn1
  CB3-1/RConn2 -- OutPhaseB1/RConn1
  Three-Phase Dynamic Load/LConn1 -- Bus_21a/LConn1
  Three-Phase Dynamic Load/LConn3 -- Bus_21a/LConn3
  Three-Phase Dynamic Load/LConn2 -- Bus_21a/LConn2

== system IEEE33BusTestSystem_DG_Control_IMC/ADN/Bus_22 ==
  Bus Load 22 : powerlib/Elements/Three-Phase Series RLC Load  LConnTagsString=A|B|C  Configuration=Y (grounded)  NominalVoltage=(12660)*v0(22)  Vabc=[1e3 1e3 1e3]  Vabcp=[1e3 1e3 1e3]  NominalFrequency=50  UnbalancedPower=off  ActivePower=90e3  InductivePower=40e3  CapacitivePower=0  Pabc=[10e3 9e3 11e3]  QLabc=[100 90 110]  QCabc=[100 90 110]  Pabcp=[10e3 9e3 11e3]  QLabcp=[100 90 110]  QCabcp=[100 90 110]  Measurements=None  LoadType=constant PQ
      settings: SourceProductName=Simscape Electrical
  Bus_22 : powerlib/Measurements/Three-Phase V-I Measurement  VoltageMeasurement=phase-to-phase  SetLabelV=on  LabelV=v22_pu  Vpu=off  VpuLL=on  CurrentMeasurement=yes  SetLabelI=on  LabelI=I2122_pu  Ipu=off  Pbase=100e6  Vbase=12660  OutputType=Complex  PhasorSimulation=on  PSBequivalent=0
      settings: SourceProductName=Simscape Electrical
  CB3-2 : powerlib/Elements/Three-Phase Breaker  InitialState=open  SwitchA=on  SwitchB=on  SwitchC=on  SwitchTimes="[1/60  5/60]"  External=on  BreakerResistance=0.01  SnubberResistance=1e6  SnubberCapacitance=inf  Measurements=None
      settings: SourceProductName=Simscape Electrical
  InPhaseA : PMIOPort  Side=Left
  InPhaseB : PMIOPort  Port=2  Side=Left
  InPhaseC : PMIOPort  Port=3  Side=Left
  OutPhaseA : PMIOPort  Port=4  Side=Right
  OutPhaseB : PMIOPort  Port=5  Side=Right
  OutPhaseC : PMIOPort  Port=6  Side=Right
  wires:
  [CB22to12] -> CB3-2/1
  connections:
  CB3-2/RConn3 -- OutPhaseC/RConn1
  Bus_22/RConn2 -- Bus Load 22/LConn2 -- CB3-2/LConn2
  Bus_22/RConn3 -- Bus Load 22/LConn3 -- CB3-2/LConn3
  CB3-2/RConn1 -- OutPhaseA/RConn1
  CB3-2/RConn2 -- OutPhaseB/RConn1
  Bus Load 22/LConn1 -- CB3-2/LConn1 -- Bus_22/RConn1
  InPhaseA/RConn1 -- Bus_22/LConn1
  InPhaseB/RConn1 -- Bus_22/LConn2
  InPhaseC/RConn1 -- Bus_22/LConn3

== system IEEE33BusTestSystem_DG_Control_IMC/ADN/Bus_23 ==
  Bus Load 23 : powerlib/Elements/Three-Phase Series RLC Load  LConnTagsString=A|B|C  Configuration=Y (grounded)  NominalVoltage=(12660)*v0(23)  Vabc=[1e3 1e3 1e3]  Vabcp=[1e3 1e3 1e3]  NominalFrequency=50  UnbalancedPower=off  ActivePower=90e3  InductivePower=50e3  CapacitivePower=0  Pabc=[10e3 9e3 11e3]  QLabc=[100 90 110]  QCabc=[100 90 110]  Pabcp=[10e3 9e3 11e3]  QLabcp=[100 90 110]  QCabcp=[100 90 110]  Measurements=None  LoadType=constant PQ
      settings: SourceProductName=Simscape Electrical
  Bus_23 : powerlib/Measurements/Three-Phase V-I Measurement  VoltageMeasurement=phase-to-phase  SetLabelV=on  LabelV=v23_pu  Vpu=off  VpuLL=on  CurrentMeasurement=yes  SetLabelI=on  LabelI=I323_pu  Ipu=off  Pbase=100e6  Vbase=12660  OutputType=Complex  PhasorSimulation=on  PSBequivalent=0
      settings: SourceProductName=Simscape Electrical
  CB3-2 : powerlib/Elements/Three-Phase Breaker  InitialState=open  SwitchA=on  SwitchB=on  SwitchC=on  SwitchTimes="[1/60  5/60]"  External=on  BreakerResistance=0.01  SnubberResistance=1e6  SnubberCapacitance=inf  Measurements=None
      settings: SourceProductName=Simscape Electrical
  InPhaseA : PMIOPort  Side=Left
  InPhaseB : PMIOPort  Port=2  Side=Left
  InPhaseC : PMIOPort  Port=3  Side=Left
  OutPhaseA : PMIOPort  Port=4  Side=Right
  OutPhaseB : PMIOPort  Port=5  Side=Right
  OutPhaseC : PMIOPort  Port=6  Side=Right
  wires:
  [CB23to24] -> CB3-2/1
  connections:
  Bus_23/RConn1 -- CB3-2/LConn1 -- Bus Load 23/LConn1
  CB3-2/RConn3 -- OutPhaseC/RConn1
  Bus Load 23/LConn2 -- CB3-2/LConn2 -- Bus_23/RConn2
  Bus Load 23/LConn3 -- CB3-2/LConn3 -- Bus_23/RConn3
  CB3-2/RConn1 -- OutPhaseA/RConn1
  CB3-2/RConn2 -- OutPhaseB/RConn1
  InPhaseA/RConn1 -- Bus_23/LConn1
  InPhaseB/RConn1 -- Bus_23/LConn2
  InPhaseC/RConn1 -- Bus_23/LConn3

== system IEEE33BusTestSystem_DG_Control_IMC/ADN/Bus_24 ==
  Bus Load 24 : powerlib/Elements/Three-Phase Series RLC Load  LConnTagsString=A|B|C  Configuration=Y (grounded)  NominalVoltage=(12660)*v0(24)  Vabc=[1e3 1e3 1e3]  Vabcp=[1e3 1e3 1e3]  NominalFrequency=50  UnbalancedPower=off  ActivePower=420e3  InductivePower=200e3  CapacitivePower=0  Pabc=[10e3 9e3 11e3]  QLabc=[100 90 110]  QCabc=[100 90 110]  Pabcp=[10e3 9e3 11e3]  QLabcp=[100 90 110]  QCabcp=[100 90 110]  Measurements=None  LoadType=constant PQ
      settings: SourceProductName=Simscape Electrical
  Bus_24 : powerlib/Measurements/Three-Phase V-I Measurement  VoltageMeasurement=phase-to-phase  SetLabelV=on  LabelV=v24_pu  Vpu=off  VpuLL=on  CurrentMeasurement=yes  SetLabelI=on  LabelI=I2324_pu  Ipu=off  Pbase=100e6  Vbase=12660  OutputType=Complex  PhasorSimulation=on  PSBequivalent=0
      settings: SourceProductName=Simscape Electrical
  CB3-2 : powerlib/Elements/Three-Phase Breaker  InitialState=open  SwitchA=on  SwitchB=on  SwitchC=on  SwitchTimes="[1/60  5/60]"  External=on  BreakerResistance=0.01  SnubberResistance=1e6  SnubberCapacitance=inf  Measurements=None
      settings: SourceProductName=Simscape Electrical
  InPhaseA : PMIOPort  Side=Left
  InPhaseB : PMIOPort  Port=2  Side=Left
  InPhaseC : PMIOPort  Port=3  Side=Left
  OutPhaseA : PMIOPort  Port=4  Side=Right
  OutPhaseB : PMIOPort  Port=5  Side=Right
  OutPhaseC : PMIOPort  Port=6  Side=Right
  wires:
  [CB24to25] -> CB3-2/1
  connections:
  Bus_24/RConn1 -- CB3-2/LConn1 -- Bus Load 24/LConn1
  CB3-2/RConn3 -- OutPhaseC/RConn1
  Bus Load 24/LConn2 -- CB3-2/LConn2 -- Bus_24/RConn2
  Bus Load 24/LConn3 -- CB3-2/LConn3 -- Bus_24/RConn3
  CB3-2/RConn1 -- OutPhaseA/RConn1
  CB3-2/RConn2 -- OutPhaseB/RConn1
  InPhaseA/RConn1 -- Bus_24/LConn1
  InPhaseB/RConn1 -- Bus_24/LConn2
  InPhaseC/RConn1 -- Bus_24/LConn3

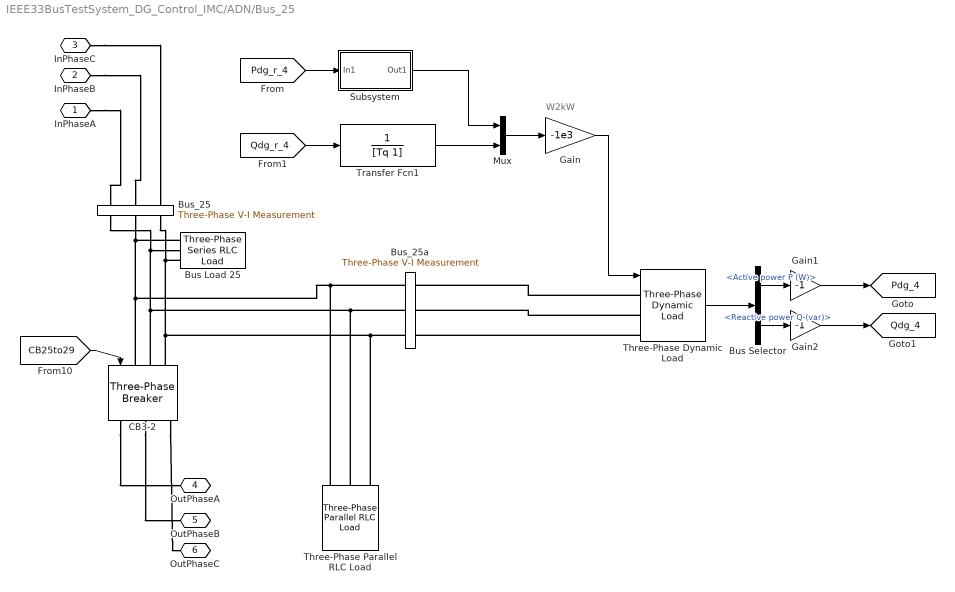
== system IEEE33BusTestSystem_DG_Control_IMC/ADN/Bus_25 ==
  note: W2kW
  Bus Load 25 : powerlib/Elements/Three-Phase Series RLC Load  LConnTagsString=A|B|C  Configuration=Y (grounded)  NominalVoltage=(12660)*v0(25)  Vabc=[1e3 1e3 1e3]  Vabcp=[1e3 1e3 1e3]  NominalFrequency=50  UnbalancedPower=off  ActivePower=420e3  InductivePower=200e3  CapacitivePower=0  Pabc=[10e3 9e3 11e3]  QLabc=[100 90 110]  QCabc=[100 90 110]  Pabcp=[10e3 9e3 11e3]  QLabcp=[100 90 110]  QCabcp=[100 90 110]  Measurements=None  LoadType=constant PQ
      settings: SourceProductName=Simscape Electrical
  Bus Selector : BusSelector  OutputSignals=Active power P (W),Reactive power Q (var)
  Bus_25 : powerlib/Measurements/Three-Phase V-I Measurement  VoltageMeasurement=phase-to-phase  SetLabelV=on  LabelV=v25_pu  Vpu=off  VpuLL=on  CurrentMeasurement=yes  SetLabelI=on  LabelI=I2425_pu  Ipu=off  Pbase=100e6  Vbase=12660  OutputType=Complex  PhasorSimulation=on  PSBequivalent=0
      settings: SourceProductName=Simscape Electrical
  Bus_25a : powerlib/Measurements/Three-Phase V-I Measurement  VoltageMeasurement=no  SetLabelV=off  LabelV=v14a_pu  Vpu=off  VpuLL=off  CurrentMeasurement=yes  SetLabelI=on  LabelI=I25a_pu  Ipu=off  Pbase=100e6  Vbase=500e3  OutputType=Complex  PhasorSimulation=on  PSBequivalent=0
      settings: SourceProductName=Simscape Electrical
  CB3-2 : powerlib/Elements/Three-Phase Breaker  InitialState=open  SwitchA=on  SwitchB=on  SwitchC=on  SwitchTimes="[1/60  5/60]"  External=on  BreakerResistance=0.01  SnubberResistance=1e6  SnubberCapacitance=inf  Measurements=None
      settings: SourceProductName=Simscape Electrical
  Gain : Gain  Gain=-1e3
  Gain1 : Gain  Gain=-1
  Gain2 : Gain  Gain=-1
  Mux : Mux  Inputs=2
  Subsystem : Subsystem
  Three-Phase Dynamic Load : powerlib/Elements/Three-Phase Dynamic Load  NominalVoltage=[ 12660 50 ]  ActiveReactivePowers=[-P_dg0(4) Q_dg0(4)]*1e3  PositiveSequence=[V_0(4) 0]  ExternalControl=on  NpNq=[1.3 2]  TimeConstants="[0  0  0  0]"  MinimumVoltage=0.7  Tfilter=1e-4  LoadFlowParameters=[4,0,0,0,0]
      settings: SourceProductName=Simscape Electrical  SourceProductBaseCode=PS
  Three-Phase Parallel RLC Load : powerlib/Elements/Three-Phase Parallel RLC Load  LConnTagsString=A|B|C  Configuration=Y (grounded)  NominalVoltage=12660  Vabc=[1e3 1e3 1e3]  Vabcp=[1e3 1e3 1e3]  NominalFrequency=50  UnbalancedPower=off  ActivePower=0.01  InductivePower=0  CapacitivePower=0  Pabc=[10e3 9e3 11e3]  QLabc=[100 90 110]  QCabc=[100 90 110]  Pabcp=[10e3 9e3 11e3]  QLabcp=[100 90 110]  QCabcp=[100 90 110]  Measurements=None  LoadType=constant Z
      settings: SourceProductName=Simscape Electrical
  Transfer Fcn1 : TransferFcn  Denominator=[Tq 1]
  InPhaseA : PMIOPort  Side=Left
  InPhaseB : PMIOPort  Port=2  Side=Left
  InPhaseC : PMIOPort  Port=3  Side=Left
  OutPhaseA : PMIOPort  Port=4  Side=Right
  OutPhaseB : PMIOPort  Port=5  Side=Right
  OutPhaseC : PMIOPort  Port=6  Side=Right
  tag scope: Pdg_4=global, Qdg_4=global
  wires:
  [CB25to29] -> CB3-2/1
  Subsystem/1(Out1) -> Mux/1
  Transfer Fcn1/1 -> Mux/2
  Bus Selector/1 -> Gain1/1  "<Active power P (W)>"
  [Pdg_r_4] -> Subsystem/1(In1)
  Gain2/1 -> [Qdg_4]
  Bus Selector/2 -> Gain2/1  "<Reactive power Q (var)>"
  Mux/1 -> Gain/1
  Three-Phase Dynamic Load/1 -> Bus Selector/1
  Gain/1 -> Three-Phase Dynamic Load/1
  Gain1/1 -> [Pdg_4]
  [Qdg_r_4] -> Transfer Fcn1/1
  connections:
  Bus_25/RConn1 -- Three-Phase Parallel RLC Load/LConn1 -- Bus_25a/RConn1 -- CB3-2/LConn1 -- Bus Load 25/LConn1
  CB3-2/RConn3 -- OutPhaseC/RConn1
  Bus Load 25/LConn2 -- Bus_25a/RConn2 -- Three-Phase Parallel RLC Load/LConn2 -- CB3-2/LConn2 -- Bus_25/RConn2
  Bus_25/RConn3 -- Three-Phase Parallel RLC Load/LConn3 -- Bus_25a/RConn3 -- CB3-2/LConn3 -- Bus Load 25/LConn3
  CB3-2/RConn1 -- OutPhaseA/RConn1
  CB3-2/RConn2 -- OutPhaseB/RConn1
  InPhaseB/RConn1 -- Bus_25/LConn2
  InPhaseA/RConn1 -- Bus_25/LConn1
  InPhaseC/RConn1 -- Bus_25/LConn3
  Three-Phase Dynamic Load/LConn1 -- Bus_25a/LConn1
  Three-Phase Dynamic Load/LConn3 -- Bus_25a/LConn3
  Three-Phase Dynamic Load/LConn2 -- Bus_25a/LConn2

== system IEEE33BusTestSystem_DG_Control_IMC/ADN/Bus_26 ==
  Bus Load 26 : powerlib/Elements/Three-Phase Series RLC Load  LConnTagsString=A|B|C  Configuration=Y (grounded)  NominalVoltage=(12660)*v0(26)  Vabc=[1e3 1e3 1e3]  Vabcp=[1e3 1e3 1e3]  NominalFrequency=50  UnbalancedPower=off  ActivePower=60e3  InductivePower=25e3  CapacitivePower=0  Pabc=[10e3 9e3 11e3]  QLabc=[100 90 110]  QCabc=[100 90 110]  Pabcp=[10e3 9e3 11e3]  QLabcp=[100 90 110]  QCabcp=[100 90 110]  Measurements=None  LoadType=constant PQ
      settings: SourceProductName=Simscape Electrical
  Bus_26 : powerlib/Measurements/Three-Phase V-I Measurement  VoltageMeasurement=phase-to-phase  SetLabelV=on  LabelV=v26_pu  Vpu=off  VpuLL=on  CurrentMeasurement=yes  SetLabelI=on  LabelI=I326_pu  Ipu=off  Pbase=100e6  Vbase=12660  OutputType=Complex  PhasorSimulation=on  PSBequivalent=0
      settings: SourceProductName=Simscape Electrical
  CB3-2 : powerlib/Elements/Three-Phase Breaker  InitialState=open  SwitchA=on  SwitchB=on  SwitchC=on  SwitchTimes="[1/60  5/60]"  External=on  BreakerResistance=0.01  SnubberResistance=1e6  SnubberCapacitance=inf  Measurements=None
      settings: SourceProductName=Simscape Electrical
  InPhaseA : PMIOPort  Side=Left
  InPhaseB : PMIOPort  Port=2  Side=Left
  InPhaseC : PMIOPort  Port=3  Side=Left
  OutPhaseA : PMIOPort  Port=4  Side=Right
  OutPhaseB : PMIOPort  Port=5  Side=Right
  OutPhaseC : PMIOPort  Port=6  Side=Right
  wires:
  [CB26to27] -> CB3-2/1
  connections:
  CB3-2/RConn3 -- OutPhaseC/RConn1
  Bus Load 26/LConn2 -- CB3-2/LConn2 -- Bus_26/RConn2
  Bus_26/RConn3 -- CB3-2/LConn3 -- Bus Load 26/LConn3
  CB3-2/RConn1 -- OutPhaseA/RConn1
  CB3-2/RConn2 -- OutPhaseB/RConn1
  Bus_26/RConn1 -- CB3-2/LConn1 -- Bus Load 26/LConn1
  InPhaseA/RConn1 -- Bus_26/LConn1
  InPhaseB/RConn1 -- Bus_26/LConn2
  InPhaseC/RConn1 -- Bus_26/LConn3

== system IEEE33BusTestSystem_DG_Control_IMC/ADN/Bus_27 ==
  Bus Load 27 : powerlib/Elements/Three-Phase Series RLC Load  LConnTagsString=A|B|C  Configuration=Y (grounded)  NominalVoltage=(12660)*v0(27)  Vabc=[1e3 1e3 1e3]  Vabcp=[1e3 1e3 1e3]  NominalFrequency=50  UnbalancedPower=off  ActivePower=60e3  InductivePower=25e3  CapacitivePower=0  Pabc=[10e3 9e3 11e3]  QLabc=[100 90 110]  QCabc=[100 90 110]  Pabcp=[10e3 9e3 11e3]  QLabcp=[100 90 110]  QCabcp=[100 90 110]  Measurements=None  LoadType=constant PQ
      settings: SourceProductName=Simscape Electrical
  Bus_27 : powerlib/Measurements/Three-Phase V-I Measurement  VoltageMeasurement=phase-to-phase  SetLabelV=on  LabelV=v27_pu  Vpu=off  VpuLL=on  CurrentMeasurement=yes  SetLabelI=on  LabelI=I2627_pu  Ipu=off  Pbase=100e6  Vbase=12660  OutputType=Complex  PhasorSimulation=on  PSBequivalent=0
      settings: SourceProductName=Simscape Electrical
  CB3-2 : powerlib/Elements/Three-Phase Breaker  InitialState=open  SwitchA=on  SwitchB=on  SwitchC=on  SwitchTimes="[1/60  5/60]"  External=on  BreakerResistance=0.01  SnubberResistance=1e6  SnubberCapacitance=inf  Measurements=None
      settings: SourceProductName=Simscape Electrical
  InPhaseA : PMIOPort  Side=Left
  InPhaseB : PMIOPort  Port=2  Side=Left
  InPhaseC : PMIOPort  Port=3  Side=Left
  OutPhaseA : PMIOPort  Port=4  Side=Right
  OutPhaseB : PMIOPort  Port=5  Side=Right
  OutPhaseC : PMIOPort  Port=6  Side=Right
  wires:
  [CB27to28] -> CB3-2/1
  connections:
  CB3-2/LConn1 -- Bus Load 27/LConn1 -- Bus_27/RConn1
  CB3-2/RConn3 -- OutPhaseC/RConn1
  CB3-2/LConn2 -- Bus Load 27/LConn2 -- Bus_27/RConn2
  Bus_27/RConn3 -- Bus Load 27/LConn3 -- CB3-2/LConn3
  CB3-2/RConn1 -- OutPhaseA/RConn1
  CB3-2/RConn2 -- OutPhaseB/RConn1
  InPhaseA/RConn1 -- Bus_27/LConn1
  InPhaseB/RConn1 -- Bus_27/LConn2
  InPhaseC/RConn1 -- Bus_27/LConn3

== system IEEE33BusTestSystem_DG_Control_IMC/ADN/Bus_28 ==
  Bus Load 28 : powerlib/Elements/Three-Phase Series RLC Load  LConnTagsString=A|B|C  Configuration=Y (grounded)  NominalVoltage=(12660)*v0(28)  Vabc=[1e3 1e3 1e3]  Vabcp=[1e3 1e3 1e3]  NominalFrequency=50  UnbalancedPower=off  ActivePower=60e3  InductivePower=20e3  CapacitivePower=0  Pabc=[10e3 9e3 11e3]  QLabc=[100 90 110]  QCabc=[100 90 110]  Pabcp=[10e3 9e3 11e3]  QLabcp=[100 90 110]  QCabcp=[100 90 110]  Measurements=None  LoadType=constant PQ
      settings: SourceProductName=Simscape Electrical
  Bus_28 : powerlib/Measurements/Three-Phase V-I Measurement  VoltageMeasurement=phase-to-phase  SetLabelV=on  LabelV=v28_pu  Vpu=off  VpuLL=on  CurrentMeasurement=yes  SetLabelI=on  LabelI=I2728_pu  Ipu=off  Pbase=100e6  Vbase=12660  OutputType=Complex  PhasorSimulation=on  PSBequivalent=0
      settings: SourceProductName=Simscape Electrical
  CB3-2 : powerlib/Elements/Three-Phase Breaker  InitialState=open  SwitchA=on  SwitchB=on  SwitchC=on  SwitchTimes="[1/60  5/60]"  External=on  BreakerResistance=0.01  SnubberResistance=1e6  SnubberCapacitance=inf  Measurements=None
      settings: SourceProductName=Simscape Electrical
  InPhaseA : PMIOPort  Side=Left
  InPhaseB : PMIOPort  Port=2  Side=Left
  InPhaseC : PMIOPort  Port=3  Side=Left
  OutPhaseA : PMIOPort  Port=4  Side=Right
  OutPhaseB : PMIOPort  Port=5  Side=Right
  OutPhaseC : PMIOPort  Port=6  Side=Right
  wires:
  [CB28to29] -> CB3-2/1
  connections:
  Bus Load 28/LConn1 -- CB3-2/LConn1 -- Bus_28/RConn1
  CB3-2/RConn3 -- OutPhaseC/RConn1
  Bus Load 28/LConn2 -- CB3-2/LConn2 -- Bus_28/RConn2
  Bus Load 28/LConn3 -- CB3-2/LConn3 -- Bus_28/RConn3
  CB3-2/RConn1 -- OutPhaseA/RConn1
  CB3-2/RConn2 -- OutPhaseB/RConn1
  InPhaseA/RConn1 -- Bus_28/LConn1
  InPhaseB/RConn1 -- Bus_28/LConn2
  InPhaseC/RConn1 -- Bus_28/LConn3

== system IEEE33BusTestSystem_DG_Control_IMC/ADN/Bus_29 ==
  Bus Load 29 : powerlib/Elements/Three-Phase Series RLC Load  LConnTagsString=A|B|C  Configuration=Y (grounded)  NominalVoltage=(12660)*v0(29)  Vabc=[1e3 1e3 1e3]  Vabcp=[1e3 1e3 1e3]  NominalFrequency=50  UnbalancedPower=off  ActivePower=120e3  InductivePower=70e3  CapacitivePower=0  Pabc=[10e3 9e3 11e3]  QLabc=[100 90 110]  QCabc=[100 90 110]  Pabcp=[10e3 9e3 11e3]  QLabcp=[100 90 110]  QCabcp=[100 90 110]  Measurements=None  LoadType=constant PQ
      settings: SourceProductName=Simscape Electrical
  Bus_29 : powerlib/Measurements/Three-Phase V-I Measurement  VoltageMeasurement=phase-to-phase  SetLabelV=on  LabelV=v29_pu  Vpu=off  VpuLL=on  CurrentMeasurement=yes  SetLabelI=on  LabelI=I2829_pu  Ipu=off  Pbase=100e6  Vbase=12660  OutputType=Complex  PhasorSimulation=on  PSBequivalent=0
      settings: SourceProductName=Simscape Electrical
  CB3-2 : powerlib/Elements/Three-Phase Breaker  InitialState=open  SwitchA=on  SwitchB=on  SwitchC=on  SwitchTimes="[1/60  5/60]"  External=on  BreakerResistance=0.01  SnubberResistance=1e6  SnubberCapacitance=inf  Measurements=None
      settings: SourceProductName=Simscape Electrical
  InPhaseA : PMIOPort  Side=Left
  InPhaseB : PMIOPort  Port=2  Side=Left
  InPhaseC : PMIOPort  Port=3  Side=Left
  OutPhaseA : PMIOPort  Port=4  Side=Right
  OutPhaseB : PMIOPort  Port=5  Side=Right
  OutPhaseC : PMIOPort  Port=6  Side=Right
  InPhaseA1 : PMIOPort  Port=7  Side=Left
  InPhaseB1 : PMIOPort  Port=8  Side=Left
  InPhaseC1 : PMIOPort  Port=9  Side=Left
  wires:
  [CB29to30] -> CB3-2/1
  connections:
  Bus_29/RConn1 -- CB3-2/LConn1 -- Bus Load 29/LConn1
  CB3-2/RConn3 -- OutPhaseC/RConn1
  Bus Load 29/LConn2 -- CB3-2/LConn2 -- Bus_29/RConn2
  Bus Load 29/LConn3 -- CB3-2/LConn3 -- Bus_29/RConn3
  CB3-2/RConn1 -- OutPhaseA/RConn1
  CB3-2/RConn2 -- OutPhaseB/RConn1
  InPhaseB1/RConn1 -- InPhaseB/RConn1 -- Bus_29/LConn2
  InPhaseA1/RConn1 -- InPhaseA/RConn1 -- Bus_29/LConn1
  InPhaseC1/RConn1 -- InPhaseC/RConn1 -- Bus_29/LConn3
